simulink model "mdl4_20160413_004644"  (R2014a)
settings: Solver=FixedStepDiscrete  SolverMode=SingleTasking  StartTime=TIME(1)  StopTime=TIME(end)  FixedStep=SIMSTEP  RelTol=1e-3
model workspace (MAT data in the model file):
  autoc_mdd_data01 : struct (value not decoded)
undefined symbols (not defined in the file): Parameter113, Parameter131, Parameter132, Parameter144, Parameter51, Parameter52, Parameter53, Parameter54, Parameter69, Parameter91, SIMSTEP
(part 2 of 3)

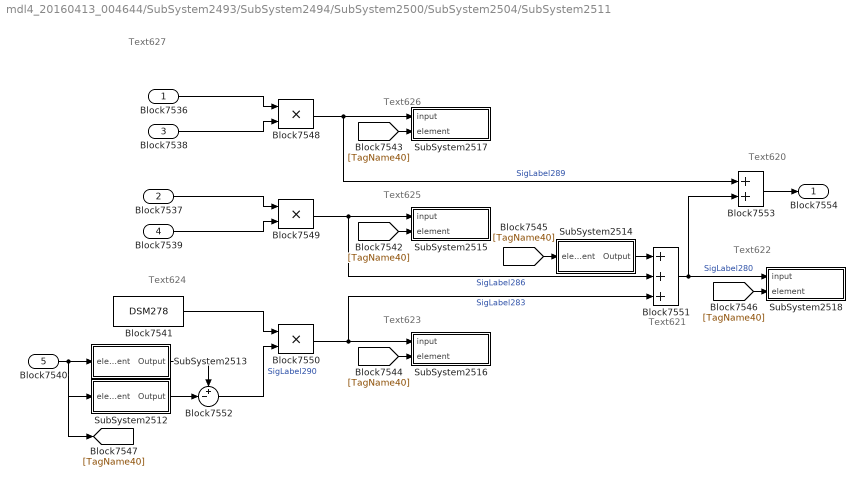
== system mdl4_20160413_004644/SubSystem2493/SubSystem2494/SubSystem2500/SubSystem2504/SubSystem2511 ==
  note: Text627
  note: Text626
  note: Text625
  note: Text624
  note: Text623
  note: Text622
  note: Text621
  note: Text620
  Block7536 : Inport
  Block7537 : Inport  Port=2
  Block7538 : Inport  Port=3
  Block7539 : Inport  Port=4
  Block7540 : Inport  Port=5
  Block7541 : DataStoreRead  DataStoreName=DSM278
  Block7548 : Product  OutDataTypeStr=double  SaturateOnIntegerOverflow=on  RndMeth=Zero  InputSameDT=on
  Block7549 : Product  OutDataTypeStr=double  SaturateOnIntegerOverflow=on  RndMeth=Zero  InputSameDT=on
  Block7550 : Product  OutDataTypeStr=double  SaturateOnIntegerOverflow=on  RndMeth=Zero  InputSameDT=on
  Block7551 : Sum  Inputs=3  OutDataTypeStr=double  RndMeth=Zero  SaturateOnIntegerOverflow=on  InputSameDT=on
  Block7552 : Sum  Inputs=+-|  OutDataTypeStr=double  RndMeth=Zero  SaturateOnIntegerOverflow=on  InputSameDT=on
  Block7553 : Sum  Inputs=2  OutDataTypeStr=double  RndMeth=Zero  SaturateOnIntegerOverflow=on  InputSameDT=on
  SubSystem2512 : Subsystem  TreatAsAtomicUnit=on  mask(***ATC.DSRVEC***){bd_version=1.01.A, r0=DSM258, r1=-1, r2=, r3=, r4=, r5=, r6=, r7=, r8=, r9=, c0=, c1=, c2=, c3=, c4=, c5=, c6=, c7=, c8=, c9=}
      mask prompts: bd_version "Version"
      mask help: これはAutoCからのブロックです．編集禁止．
      settings: OpenFcn=warndlg('変更禁止!');
      mask Help: web(ui_blockhelpmng(gcb));
      mask Display: disp('ATC.DSRVEC')
  SubSystem2513 : Subsystem  TreatAsAtomicUnit=on  mask(***ATC.DSRVEC***){bd_version=1.01.A, r0=DSM259, r1=-1, r2=, r3=, r4=, r5=, r6=, r7=, r8=, r9=, c0=, c1=, c2=, c3=, c4=, c5=, c6=, c7=, c8=, c9=}
      mask prompts: bd_version "Version"
      mask help: これはAutoCからのブロックです．編集禁止．
      settings: OpenFcn=warndlg('変更禁止!');
      mask Help: web(ui_blockhelpmng(gcb));
      mask Display: disp('ATC.DSRVEC')
  SubSystem2514 : Subsystem  TreatAsAtomicUnit=on  mask(***ATC.DSRVEC***){bd_version=1.01.A, r0=DSM300, r1=-1, r2=, r3=, r4=, r5=, r6=, r7=, r8=, r9=, c0=, c1=, c2=, c3=, c4=, c5=, c6=, c7=, c8=, c9=}
      mask prompts: bd_version "Version"
      mask help: これはAutoCからのブロックです．編集禁止．
      settings: OpenFcn=warndlg('変更禁止!');
      mask Help: web(ui_blockhelpmng(gcb));
      mask Display: disp('ATC.DSRVEC')
  SubSystem2515 : Subsystem  TreatAsAtomicUnit=on  mask(***ATC.DSWVEC***){bd_version=1.01.A, r0=DSM302, r1=-1, r2=, r3=, r4=, r5=, r6=, r7=, r8=, r9=, c0=, c1=, c2=, c3=, c4=, c5=, c6=, c7=, c8=, c9=}
      mask prompts: bd_version "Version"
      mask help: これはAutoCからのブロックです．編集禁止．
      settings: OpenFcn=warndlg('変更禁止!');
      mask Help: web(ui_blockhelpmng(gcb));
      mask Display: disp('ATC.DSRVEC')
  SubSystem2516 : Subsystem  TreatAsAtomicUnit=on  mask(***ATC.DSWVEC***){bd_version=1.01.A, r0=DSM301, r1=-1, r2=, r3=, r4=, r5=, r6=, r7=, r8=, r9=, c0=, c1=, c2=, c3=, c4=, c5=, c6=, c7=, c8=, c9=}
      mask prompts: bd_version "Version"
      mask help: これはAutoCからのブロックです．編集禁止．
      settings: OpenFcn=warndlg('変更禁止!');
      mask Help: web(ui_blockhelpmng(gcb));
      mask Display: disp('ATC.DSRVEC')
  SubSystem2517 : Subsystem  TreatAsAtomicUnit=on  mask(***ATC.DSWVEC***){bd_version=1.01.A, r0=DSM303, r1=-1, r2=, r3=, r4=, r5=, r6=, r7=, r8=, r9=, c0=, c1=, c2=, c3=, c4=, c5=, c6=, c7=, c8=, c9=}
      mask prompts: bd_version "Version"
      mask help: これはAutoCからのブロックです．編集禁止．
      settings: OpenFcn=warndlg('変更禁止!');
      mask Help: web(ui_blockhelpmng(gcb));
      mask Display: disp('ATC.DSRVEC')
  SubSystem2518 : Subsystem  TreatAsAtomicUnit=on  mask(***ATC.DSWVEC***){bd_version=1.01.A, r0=DSM300, r1=-1, r2=, r3=, r4=, r5=, r6=, r7=, r8=, r9=, c0=, c1=, c2=, c3=, c4=, c5=, c6=, c7=, c8=, c9=}
      mask prompts: bd_version "Version"
      mask help: これはAutoCからのブロックです．編集禁止．
      settings: OpenFcn=warndlg('変更禁止!');
      mask Help: web(ui_blockhelpmng(gcb));
      mask Display: disp('ATC.DSRVEC')
  Block7554 : Outport
  wires:
  SubSystem2512/1(Output) -> Block7552/2
  SubSystem2513/1(Output) -> Block7552/1
  Block7540/1 -> SubSystem2513/1(element), SubSystem2512/1(element), [TagName40]
  Block7552/1 -> Block7550/2  "SigLabel290"
  Block7548/1 -> SubSystem2517/1(input), Block7553/1  "SigLabel289"
  [TagName40] -> SubSystem2517/2(element)
  Block7549/1 -> SubSystem2515/1(input), Block7551/2  "SigLabel286"
  [TagName40] -> SubSystem2515/2(element)
  Block7541/1 -> Block7550/1
  Block7550/1 -> SubSystem2516/1(input), Block7551/3  "SigLabel283"
  [TagName40] -> SubSystem2516/2(element)
  [TagName40] -> SubSystem2514/1(element)
  [TagName40] -> SubSystem2518/2(element)
  SubSystem2514/1(Output) -> Block7551/1
  Block7551/1 -> SubSystem2518/1(input), Block7553/2  "SigLabel280"
  Block7553/1 -> Block7554/1
  Block7536/1 -> Block7548/1
  Block7538/1 -> Block7548/2
  Block7537/1 -> Block7549/1
  Block7539/1 -> Block7549/2

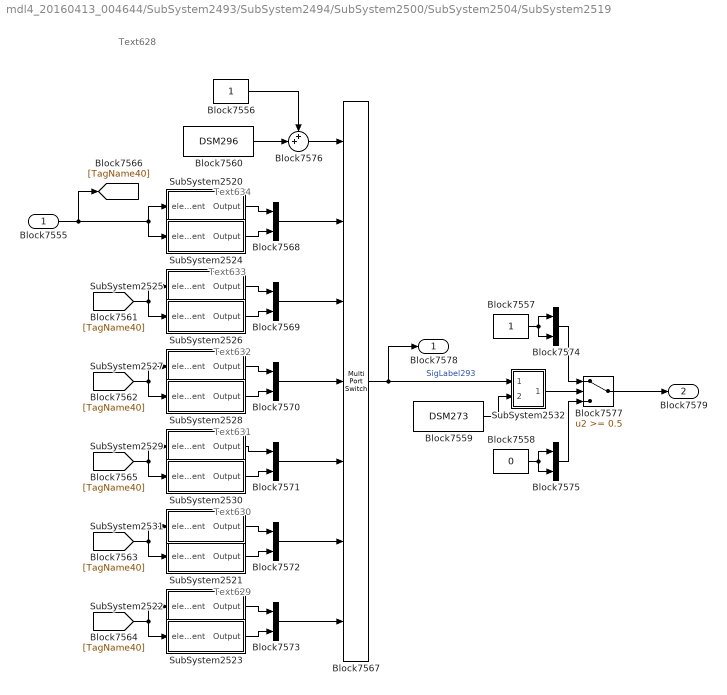
== system mdl4_20160413_004644/SubSystem2493/SubSystem2494/SubSystem2500/SubSystem2504/SubSystem2519 ==
  note: Text634
  note: Text633
  note: Text632
  note: Text631
  note: Text630
  note: Text629
  note: Text628
  Block7555 : Inport
  Block7556 : Constant  OutDataTypeStr=double  SampleTime=-1
  Block7557 : Constant  OutDataTypeStr=double  SampleTime=-1
  Block7558 : Constant  Value=0  OutDataTypeStr=double  SampleTime=-1
  Block7559 : DataStoreRead  DataStoreName=DSM273
  Block7560 : DataStoreRead  DataStoreName=DSM296
  Block7567 : MultiPortSwitch  Inputs=6  RndMeth=Zero  SaturateOnIntegerOverflow=on  InputSameDT=on
  Block{7568..7575} (8 alike) : Mux  Inputs=2
  Block7576 : Sum  Inputs=++|  OutDataTypeStr=double  RndMeth=Zero  SaturateOnIntegerOverflow=on  InputSameDT=on
  Block7577 : Switch  Threshold=0.5  RndMeth=Zero  SaturateOnIntegerOverflow=on  InputSameDT=on
  SubSystem2520 : Subsystem  TreatAsAtomicUnit=on  mask(***ATC.DSRVEC***){bd_version=1.01.A, r0=DSM114, r1=-1, r2=, r3=, r4=, r5=, r6=, r7=, r8=, r9=, c0=, c1=, c2=, c3=, c4=, c5=, c6=, c7=, c8=, c9=}
      mask prompts: bd_version "Version"
      mask help: これはAutoCからのブロックです．編集禁止．
      settings: OpenFcn=warndlg('変更禁止!');
      mask Help: web(ui_blockhelpmng(gcb));
      mask Display: disp('ATC.DSRVEC')
  SubSystem2521 : Subsystem  TreatAsAtomicUnit=on  mask(***ATC.DSRVEC***){bd_version=1.01.A, r0=DSM105, r1=-1, r2=, r3=, r4=, r5=, r6=, r7=, r8=, r9=, c0=, c1=, c2=, c3=, c4=, c5=, c6=, c7=, c8=, c9=}
      mask prompts: bd_version "Version"
      mask help: これはAutoCからのブロックです．編集禁止．
      settings: OpenFcn=warndlg('変更禁止!');
      mask Help: web(ui_blockhelpmng(gcb));
      mask Display: disp('ATC.DSRVEC')
  SubSystem2522 : Subsystem  TreatAsAtomicUnit=on  mask(***ATC.DSRVEC***){bd_version=1.01.A, r0=DSM111, r1=-1, r2=, r3=, r4=, r5=, r6=, r7=, r8=, r9=, c0=, c1=, c2=, c3=, c4=, c5=, c6=, c7=, c8=, c9=}
      mask prompts: bd_version "Version"
      mask help: これはAutoCからのブロックです．編集禁止．
      settings: OpenFcn=warndlg('変更禁止!');
      mask Help: web(ui_blockhelpmng(gcb));
      mask Display: disp('ATC.DSRVEC')
  SubSystem2523 : Subsystem  TreatAsAtomicUnit=on  mask(***ATC.DSRVEC***){bd_version=1.01.A, r0=DSM113, r1=-1, r2=, r3=, r4=, r5=, r6=, r7=, r8=, r9=, c0=, c1=, c2=, c3=, c4=, c5=, c6=, c7=, c8=, c9=}
      mask prompts: bd_version "Version"
      mask help: これはAutoCからのブロックです．編集禁止．
      settings: OpenFcn=warndlg('変更禁止!');
      mask Help: web(ui_blockhelpmng(gcb));
      mask Display: disp('ATC.DSRVEC')
  SubSystem2524 : Subsystem  TreatAsAtomicUnit=on  mask(***ATC.DSRVEC***){bd_version=1.01.A, r0=DSM118, r1=-1, r2=, r3=, r4=, r5=, r6=, r7=, r8=, r9=, c0=, c1=, c2=, c3=, c4=, c5=, c6=, c7=, c8=, c9=}
      mask prompts: bd_version "Version"
      mask help: これはAutoCからのブロックです．編集禁止．
      settings: OpenFcn=warndlg('変更禁止!');
      mask Help: web(ui_blockhelpmng(gcb));
      mask Display: disp('ATC.DSRVEC')
  SubSystem2525 : Subsystem  TreatAsAtomicUnit=on  mask(***ATC.DSRVEC***){bd_version=1.01.A, r0=DSM117, r1=-1, r2=, r3=, r4=, r5=, r6=, r7=, r8=, r9=, c0=, c1=, c2=, c3=, c4=, c5=, c6=, c7=, c8=, c9=}
      mask prompts: bd_version "Version"
      mask help: これはAutoCからのブロックです．編集禁止．
      settings: OpenFcn=warndlg('変更禁止!');
      mask Help: web(ui_blockhelpmng(gcb));
      mask Display: disp('ATC.DSRVEC')
  SubSystem2526 : Subsystem  TreatAsAtomicUnit=on  mask(***ATC.DSRVEC***){bd_version=1.01.A, r0=DSM121, r1=-1, r2=, r3=, r4=, r5=, r6=, r7=, r8=, r9=, c0=, c1=, c2=, c3=, c4=, c5=, c6=, c7=, c8=, c9=}
      mask prompts: bd_version "Version"
      mask help: これはAutoCからのブロックです．編集禁止．
      settings: OpenFcn=warndlg('変更禁止!');
      mask Help: web(ui_blockhelpmng(gcb));
      mask Display: disp('ATC.DSRVEC')
  SubSystem2527 : Subsystem  TreatAsAtomicUnit=on  mask(***ATC.DSRVEC***){bd_version=1.01.A, r0=DSM124, r1=-1, r2=, r3=, r4=, r5=, r6=, r7=, r8=, r9=, c0=, c1=, c2=, c3=, c4=, c5=, c6=, c7=, c8=, c9=}
      mask prompts: bd_version "Version"
      mask help: これはAutoCからのブロックです．編集禁止．
      settings: OpenFcn=warndlg('変更禁止!');
      mask Help: web(ui_blockhelpmng(gcb));
      mask Display: disp('ATC.DSRVEC')
  SubSystem2528 : Subsystem  TreatAsAtomicUnit=on  mask(***ATC.DSRVEC***){bd_version=1.01.A, r0=DSM127, r1=-1, r2=, r3=, r4=, r5=, r6=, r7=, r8=, r9=, c0=, c1=, c2=, c3=, c4=, c5=, c6=, c7=, c8=, c9=}
      mask prompts: bd_version "Version"
      mask help: これはAutoCからのブロックです．編集禁止．
      settings: OpenFcn=warndlg('変更禁止!');
      mask Help: web(ui_blockhelpmng(gcb));
      mask Display: disp('ATC.DSRVEC')
  SubSystem2529 : Subsystem  TreatAsAtomicUnit=on  mask(***ATC.DSRVEC***){bd_version=1.01.A, r0=DSM107, r1=-1, r2=, r3=, r4=, r5=, r6=, r7=, r8=, r9=, c0=, c1=, c2=, c3=, c4=, c5=, c6=, c7=, c8=, c9=}
      mask prompts: bd_version "Version"
      mask help: これはAutoCからのブロックです．編集禁止．
      settings: OpenFcn=warndlg('変更禁止!');
      mask Help: web(ui_blockhelpmng(gcb));
      mask Display: disp('ATC.DSRVEC')
  SubSystem2530 : Subsystem  TreatAsAtomicUnit=on  mask(***ATC.DSRVEC***){bd_version=1.01.A, r0=DSM109, r1=-1, r2=, r3=, r4=, r5=, r6=, r7=, r8=, r9=, c0=, c1=, c2=, c3=, c4=, c5=, c6=, c7=, c8=, c9=}
      mask prompts: bd_version "Version"
      mask help: これはAutoCからのブロックです．編集禁止．
      settings: OpenFcn=warndlg('変更禁止!');
      mask Help: web(ui_blockhelpmng(gcb));
      mask Display: disp('ATC.DSRVEC')
  SubSystem2531 : Subsystem  TreatAsAtomicUnit=on  mask(***ATC.DSRVEC***){bd_version=1.01.A, r0=DSM103, r1=-1, r2=, r3=, r4=, r5=, r6=, r7=, r8=, r9=, c0=, c1=, c2=, c3=, c4=, c5=, c6=, c7=, c8=, c9=}
      mask prompts: bd_version "Version"
      mask help: これはAutoCからのブロックです．編集禁止．
      settings: OpenFcn=warndlg('変更禁止!');
      mask Help: web(ui_blockhelpmng(gcb));
      mask Display: disp('ATC.DSRVEC')
  SubSystem2532 : Subsystem
  Block7578 : Outport
  Block7579 : Outport  Port=2
  wires:
  Block7560/1 -> Block7576/2
  Block7556/1 -> Block7576/1
  Block7576/1 -> Block7567/1
  Block7555/1 -> SubSystem2524/1(element), SubSystem2520/1(element), [TagName40]
  SubSystem2520/1(Output) -> Block7568/1
  SubSystem2524/1(Output) -> Block7568/2
  Block7568/1 -> Block7567/2
  [TagName40] -> SubSystem2525/1(element), SubSystem2526/1(element)
  SubSystem2525/1(Output) -> Block7569/1
  SubSystem2526/1(Output) -> Block7569/2
  [TagName40] -> SubSystem2527/1(element), SubSystem2528/1(element)
  SubSystem2527/1(Output) -> Block7570/1
  SubSystem2528/1(Output) -> Block7570/2
  [TagName40] -> SubSystem2529/1(element), SubSystem2530/1(element)
  SubSystem2530/1(Output) -> Block7571/2
  [TagName40] -> SubSystem2531/1(element), SubSystem2521/1(element)
  SubSystem2531/1(Output) -> Block7572/1
  SubSystem2521/1(Output) -> Block7572/2
  [TagName40] -> SubSystem2522/1(element), SubSystem2523/1(element)
  SubSystem2522/1(Output) -> Block7573/1
  SubSystem2523/1(Output) -> Block7573/2
  SubSystem2529/1(Output) -> Block7571/1
  Block7569/1 -> Block7567/3
  Block7570/1 -> Block7567/4
  Block7571/1 -> Block7567/5
  Block7572/1 -> Block7567/6
  Block7573/1 -> Block7567/7
  Block7567/1 -> Block7578/1, SubSystem2532/1(In1)  "SigLabel293"
  Block7559/1 -> SubSystem2532/2(In2)
  SubSystem2532/1(Out1) -> Block7577/2
  Block7577/1 -> Block7579/1
  Block7557/1 -> Block7574/1, Block7574/2
  Block7558/1 -> Block7575/1, Block7575/2
  Block7574/1 -> Block7577/1
  Block7575/1 -> Block7577/3

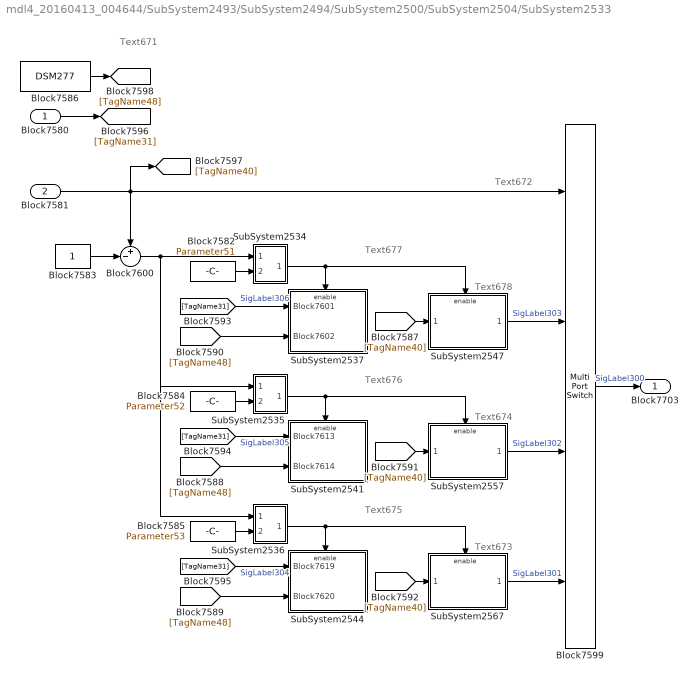
== system mdl4_20160413_004644/SubSystem2493/SubSystem2494/SubSystem2500/SubSystem2504/SubSystem2533 ==
  note: Text678
  note: Text677
  note: Text676
  note: Text675
  note: Text674
  note: Text673
  note: Text672
  note: Text671
  Block7580 : Inport
  Block7581 : Inport  Port=2
  Block7582 : Constant  Value=Parameter51  OutDataTypeStr=double  SampleTime=-1
  Block7583 : Constant  OutDataTypeStr=double  SampleTime=-1
  Block7584 : Constant  Value=Parameter52  OutDataTypeStr=double  SampleTime=-1
  Block7585 : Constant  Value=Parameter53  OutDataTypeStr=double  SampleTime=-1
  Block7586 : DataStoreRead  DataStoreName=DSM277
  Block7599 : MultiPortSwitch  RndMeth=Zero  SaturateOnIntegerOverflow=on  InputSameDT=on
  Block7600 : Sum  Inputs=+-|  OutDataTypeStr=double  RndMeth=Zero  SaturateOnIntegerOverflow=on  InputSameDT=on
  SubSystem2534 : Subsystem
  SubSystem2535 : Subsystem
  SubSystem2536 : Subsystem
  SubSystem2537 : Subsystem  Priority=10  TreatAsAtomicUnit=on
      settings: AttributesFormatString=Attribute1933
  SubSystem2541 : Subsystem  Priority=10  TreatAsAtomicUnit=on
      settings: AttributesFormatString=Attribute1939
  SubSystem2544 : Subsystem  Priority=10  TreatAsAtomicUnit=on
      settings: AttributesFormatString=Attribute1943
  SubSystem2547 : Subsystem  Priority=20  TreatAsAtomicUnit=on
      settings: AttributesFormatString=Attribute1947
  SubSystem2557 : Subsystem  Priority=20  TreatAsAtomicUnit=on
      settings: AttributesFormatString=Attribute1954
  SubSystem2567 : Subsystem  Priority=20  TreatAsAtomicUnit=on
      settings: AttributesFormatString=Attribute1961
  Block7703 : Outport
  wires:
  Block7582/1 -> SubSystem2534/2(In2)
  SubSystem2534/1(Out1) -> SubSystem2537/Enable, SubSystem2547/Enable
  [TagName31] -> SubSystem2537/1(Block7601)  "SigLabel306"
  Block7584/1 -> SubSystem2535/2(In2)
  [TagName48] -> SubSystem2541/2(Block7614)
  SubSystem2535/1(Out1) -> SubSystem2541/Enable, SubSystem2557/Enable
  [TagName31] -> SubSystem2541/1(Block7613)  "SigLabel305"
  Block7585/1 -> SubSystem2536/2(In2)
  [TagName48] -> SubSystem2544/2(Block7620)
  SubSystem2536/1(Out1) -> SubSystem2544/Enable, SubSystem2567/Enable
  [TagName31] -> SubSystem2544/1(Block7619)  "SigLabel304"
  [TagName48] -> SubSystem2537/2(Block7602)
  SubSystem2547/1(Block7650) -> Block7599/2  "SigLabel303"
  SubSystem2557/1(Block7676) -> Block7599/3  "SigLabel302"
  SubSystem2567/1(Block7702) -> Block7599/4  "SigLabel301"
  Block7581/1 -> Block7599/1, Block7600/1, [TagName40]
  Block7599/1 -> Block7703/1  "SigLabel300"
  Block7583/1 -> Block7600/2
  Block7600/1 -> SubSystem2535/1(In1), SubSystem2536/1(In1), SubSystem2534/1(In1)
  Block7586/1 -> [TagName48]
  Block7580/1 -> [TagName31]
  [TagName40] -> SubSystem2547/1(Block7625)
  [TagName40] -> SubSystem2557/1(Block7651)
  [TagName40] -> SubSystem2567/1(Block7677)

== system mdl4_20160413_004644/SubSystem2493/SubSystem2577/SubSystem2579/SubSystem2581/SubSystem2582 ==
  note: ***編集禁止***
  input : Inport
  element : Inport  Port=2
  Assignment : Assignment  IndexOptions=Index vector (port)  OutputSizes=[1 1]
  Inside_DSR : DataStoreRead  DataStoreName=DSM258
  Inside_DSW : DataStoreWrite  DataStoreName=DSM258
  wires:
  Assignment/1 -> Inside_DSW/1
  Inside_DSR/1 -> Assignment/1
  input/1 -> Assignment/2
  element/1 -> Assignment/3

== system mdl4_20160413_004644/SubSystem2493/SubSystem2577/SubSystem2579/SubSystem2581/SubSystem2583 ==
  note: ***編集禁止***
  input : Inport
  element : Inport  Port=2
  Assignment : Assignment  IndexOptions=Index vector (port)  OutputSizes=[1 1]
  Inside_DSR : DataStoreRead  DataStoreName=DSM275
  Inside_DSW : DataStoreWrite  DataStoreName=DSM275
  wires:
  Assignment/1 -> Inside_DSW/1
  Inside_DSR/1 -> Assignment/1
  input/1 -> Assignment/2
  element/1 -> Assignment/3

== system mdl4_20160413_004644/SubSystem2493/SubSystem2577/SubSystem2579/SubSystem2581/SubSystem2584 ==
  note: ***編集禁止***
  input : Inport
  element : Inport  Port=2
  Assignment : Assignment  IndexOptions=Index vector (port)  OutputSizes=[1 1]
  Inside_DSR : DataStoreRead  DataStoreName=DSM295
  Inside_DSW : DataStoreWrite  DataStoreName=DSM295
  wires:
  Assignment/1 -> Inside_DSW/1
  Inside_DSR/1 -> Assignment/1
  input/1 -> Assignment/2
  element/1 -> Assignment/3

== system mdl4_20160413_004644/SubSystem2493/SubSystem2577/SubSystem2579/SubSystem2581/SubSystem2585 ==
  note: ***編集禁止***
  input : Inport
  element : Inport  Port=2
  Assignment : Assignment  IndexOptions=Index vector (port)  OutputSizes=[1 1]
  Inside_DSR : DataStoreRead  DataStoreName=DSM280
  Inside_DSW : DataStoreWrite  DataStoreName=DSM280
  wires:
  Assignment/1 -> Inside_DSW/1
  Inside_DSR/1 -> Assignment/1
  input/1 -> Assignment/2
  element/1 -> Assignment/3

== system mdl4_20160413_004644/SubSystem2493/SubSystem2577/SubSystem2579/SubSystem2581/SubSystem2586 ==
  note: ***編集禁止***
  input : Inport
  element : Inport  Port=2
  Assignment : Assignment  IndexOptions=Index vector (port)  OutputSizes=[1 1]
  Inside_DSR : DataStoreRead  DataStoreName=DSM282
  Inside_DSW : DataStoreWrite  DataStoreName=DSM282
  wires:
  Assignment/1 -> Inside_DSW/1
  Inside_DSR/1 -> Assignment/1
  input/1 -> Assignment/2
  element/1 -> Assignment/3

== system mdl4_20160413_004644/SubSystem2493/SubSystem2577/SubSystem2579/SubSystem2581/SubSystem2587 ==
  note: ***編集禁止***
  input : Inport
  element : Inport  Port=2
  Assignment : Assignment  IndexOptions=Index vector (port)  OutputSizes=[1 1]
  Inside_DSR : DataStoreRead  DataStoreName=DSM274
  Inside_DSW : DataStoreWrite  DataStoreName=DSM274
  wires:
  Assignment/1 -> Inside_DSW/1
  Inside_DSR/1 -> Assignment/1
  input/1 -> Assignment/2
  element/1 -> Assignment/3

== system mdl4_20160413_004644/SubSystem2493/SubSystem2577/SubSystem2579/SubSystem2581/SubSystem2588 ==
  note: ***編集禁止***
  input : Inport
  element : Inport  Port=2
  Assignment : Assignment  IndexOptions=Index vector (port)  OutputSizes=[1 1]
  Inside_DSR : DataStoreRead  DataStoreName=DSM302
  Inside_DSW : DataStoreWrite  DataStoreName=DSM302
  wires:
  Assignment/1 -> Inside_DSW/1
  Inside_DSR/1 -> Assignment/1
  input/1 -> Assignment/2
  element/1 -> Assignment/3

== system mdl4_20160413_004644/SubSystem2493/SubSystem2577/SubSystem2579/SubSystem2581/SubSystem2589 ==
  note: ***編集禁止***
  input : Inport
  element : Inport  Port=2
  Assignment : Assignment  IndexOptions=Index vector (port)  OutputSizes=[1 1]
  Inside_DSR : DataStoreRead  DataStoreName=DSM303
  Inside_DSW : DataStoreWrite  DataStoreName=DSM303
  wires:
  Assignment/1 -> Inside_DSW/1
  Inside_DSR/1 -> Assignment/1
  input/1 -> Assignment/2
  element/1 -> Assignment/3

== system mdl4_20160413_004644/SubSystem2493/SubSystem2577/SubSystem2579/SubSystem2581/SubSystem2590 ==
  note: ***編集禁止***
  input : Inport
  element : Inport  Port=2
  Assignment : Assignment  IndexOptions=Index vector (port)  OutputSizes=[1 1]
  Inside_DSR : DataStoreRead  DataStoreName=DSM300
  Inside_DSW : DataStoreWrite  DataStoreName=DSM300
  wires:
  Assignment/1 -> Inside_DSW/1
  Inside_DSR/1 -> Assignment/1
  input/1 -> Assignment/2
  element/1 -> Assignment/3

== system mdl4_20160413_004644/SubSystem2493/SubSystem2577/SubSystem2579/SubSystem2581/SubSystem2591 ==
  note: ***編集禁止***
  input : Inport
  element : Inport  Port=2
  Assignment : Assignment  IndexOptions=Index vector (port)  OutputSizes=[1 1]
  Inside_DSR : DataStoreRead  DataStoreName=DSM301
  Inside_DSW : DataStoreWrite  DataStoreName=DSM301
  wires:
  Assignment/1 -> Inside_DSW/1
  Inside_DSR/1 -> Assignment/1
  input/1 -> Assignment/2
  element/1 -> Assignment/3

== system mdl4_20160413_004644/SubSystem2493/SubSystem2577/SubSystem2579/SubSystem2581/SubSystem2592 ==
  note: ***編集禁止***
  input : Inport
  element : Inport  Port=2
  Assignment : Assignment  IndexOptions=Index vector (port)  OutputSizes=[1 1]
  Inside_DSR : DataStoreRead  DataStoreName=DSM293
  Inside_DSW : DataStoreWrite  DataStoreName=DSM293
  wires:
  Assignment/1 -> Inside_DSW/1
  Inside_DSR/1 -> Assignment/1
  input/1 -> Assignment/2
  element/1 -> Assignment/3

== system mdl4_20160413_004644/SubSystem2493/SubSystem2577/SubSystem2579/SubSystem2581/SubSystem2593 ==
  note: ***編集禁止***
  input : Inport
  element : Inport  Port=2
  Assignment : Assignment  IndexOptions=Index vector (port)  OutputSizes=[1 1]
  Inside_DSR : DataStoreRead  DataStoreName=DSM279
  Inside_DSW : DataStoreWrite  DataStoreName=DSM279
  wires:
  Assignment/1 -> Inside_DSW/1
  Inside_DSR/1 -> Assignment/1
  input/1 -> Assignment/2
  element/1 -> Assignment/3

== system mdl4_20160413_004644/SubSystem2493/SubSystem2577/SubSystem2579/SubSystem2581/SubSystem2594 ==
  note: ***編集禁止***
  input : Inport
  element : Inport  Port=2
  Assignment : Assignment  IndexOptions=Index vector (port)  OutputSizes=[1 1]
  Inside_DSR : DataStoreRead  DataStoreName=DSM281
  Inside_DSW : DataStoreWrite  DataStoreName=DSM281
  wires:
  Assignment/1 -> Inside_DSW/1
  Inside_DSR/1 -> Assignment/1
  input/1 -> Assignment/2
  element/1 -> Assignment/3

== system mdl4_20160413_004644/SubSystem2493/SubSystem2494/SubSystem2500/SubSystem2504/SubSystem2507/SubSystem2508 ==
  note: ***編集禁止***
  In1 : Inport
  In2 : Inport  Port=2
  RO1 : RelationalOperator  Operator===  InputSameDT=on
  single1 : DataTypeConversion  OutDataTypeStr=single  SaturateOnIntegerOverflow=on  RndMeth=Zero
  single2 : DataTypeConversion  OutDataTypeStr=single  SaturateOnIntegerOverflow=on  RndMeth=Zero
  Out1 : Outport
  wires:
  RO1/1 -> Out1/1
  In2/1 -> single2/1
  In1/1 -> single1/1
  single1/1 -> RO1/1
  single2/1 -> RO1/2

== system mdl4_20160413_004644/SubSystem2493/SubSystem2494/SubSystem2500/SubSystem2504/SubSystem2509/SubSystem2510 ==
  note: ***編集禁止***
  In1 : Inport
  In2 : Inport  Port=2
  RO1 : RelationalOperator  Operator===  InputSameDT=on
  single1 : DataTypeConversion  OutDataTypeStr=single  SaturateOnIntegerOverflow=on  RndMeth=Zero
  single2 : DataTypeConversion  OutDataTypeStr=single  SaturateOnIntegerOverflow=on  RndMeth=Zero
  Out1 : Outport
  wires:
  single2/1 -> RO1/2
  single1/1 -> RO1/1
  In1/1 -> single1/1
  In2/1 -> single2/1
  RO1/1 -> Out1/1

== system mdl4_20160413_004644/SubSystem2493/SubSystem2494/SubSystem2500/SubSystem2504/SubSystem2511/SubSystem2512 ==
  note: ***編集禁止***
  element : Inport
  Inside_DSR : DataStoreRead  DataStoreName=DSM258
  Selector : Selector  IndexOptions=Index vector (port)  Indices=[1 3]
  Output : Outport
  wires:
  Inside_DSR/1 -> Selector/1
  element/1 -> Selector/2
  Selector/1 -> Output/1

== system mdl4_20160413_004644/SubSystem2493/SubSystem2494/SubSystem2500/SubSystem2504/SubSystem2511/SubSystem2513 ==
  note: ***編集禁止***
  element : Inport
  Inside_DSR : DataStoreRead  DataStoreName=DSM259
  Selector : Selector  IndexOptions=Index vector (port)  Indices=[1 3]
  Output : Outport
  wires:
  Selector/1 -> Output/1
  element/1 -> Selector/2
  Inside_DSR/1 -> Selector/1

== system mdl4_20160413_004644/SubSystem2493/SubSystem2494/SubSystem2500/SubSystem2504/SubSystem2511/SubSystem2514 ==
  note: ***編集禁止***
  element : Inport
  Inside_DSR : DataStoreRead  DataStoreName=DSM300
  Selector : Selector  IndexOptions=Index vector (port)  Indices=[1 3]
  Output : Outport
  wires:
  Inside_DSR/1 -> Selector/1
  element/1 -> Selector/2
  Selector/1 -> Output/1

== system mdl4_20160413_004644/SubSystem2493/SubSystem2494/SubSystem2500/SubSystem2504/SubSystem2511/SubSystem2515 ==
  note: ***編集禁止***
  input : Inport
  element : Inport  Port=2
  Assignment : Assignment  IndexOptions=Index vector (port)  OutputSizes=[1 1]
  Inside_DSR : DataStoreRead  DataStoreName=DSM302
  Inside_DSW : DataStoreWrite  DataStoreName=DSM302
  wires:
  element/1 -> Assignment/3
  input/1 -> Assignment/2
  Inside_DSR/1 -> Assignment/1
  Assignment/1 -> Inside_DSW/1

== system mdl4_20160413_004644/SubSystem2493/SubSystem2494/SubSystem2500/SubSystem2504/SubSystem2511/SubSystem2516 ==
  note: ***編集禁止***
  input : Inport
  element : Inport  Port=2
  Assignment : Assignment  IndexOptions=Index vector (port)  OutputSizes=[1 1]
  Inside_DSR : DataStoreRead  DataStoreName=DSM301
  Inside_DSW : DataStoreWrite  DataStoreName=DSM301
  wires:
  Assignment/1 -> Inside_DSW/1
  Inside_DSR/1 -> Assignment/1
  input/1 -> Assignment/2
  element/1 -> Assignment/3

== system mdl4_20160413_004644/SubSystem2493/SubSystem2494/SubSystem2500/SubSystem2504/SubSystem2511/SubSystem2517 ==
  note: ***編集禁止***
  input : Inport
  element : Inport  Port=2
  Assignment : Assignment  IndexOptions=Index vector (port)  OutputSizes=[1 1]
  Inside_DSR : DataStoreRead  DataStoreName=DSM303
  Inside_DSW : DataStoreWrite  DataStoreName=DSM303
  wires:
  Assignment/1 -> Inside_DSW/1
  Inside_DSR/1 -> Assignment/1
  input/1 -> Assignment/2
  element/1 -> Assignment/3

== system mdl4_20160413_004644/SubSystem2493/SubSystem2494/SubSystem2500/SubSystem2504/SubSystem2511/SubSystem2518 ==
  note: ***編集禁止***
  input : Inport
  element : Inport  Port=2
  Assignment : Assignment  IndexOptions=Index vector (port)  OutputSizes=[1 1]
  Inside_DSR : DataStoreRead  DataStoreName=DSM300
  Inside_DSW : DataStoreWrite  DataStoreName=DSM300
  wires:
  element/1 -> Assignment/3
  input/1 -> Assignment/2
  Inside_DSR/1 -> Assignment/1
  Assignment/1 -> Inside_DSW/1

== system mdl4_20160413_004644/SubSystem2493/SubSystem2494/SubSystem2500/SubSystem2504/SubSystem2519/SubSystem2520 ==
  note: ***編集禁止***
  element : Inport
  Inside_DSR : DataStoreRead  DataStoreName=DSM114
  Selector : Selector  IndexOptions=Index vector (port)  Indices=[1 3]
  Output : Outport
  wires:
  Inside_DSR/1 -> Selector/1
  element/1 -> Selector/2
  Selector/1 -> Output/1

== system mdl4_20160413_004644/SubSystem2493/SubSystem2494/SubSystem2500/SubSystem2504/SubSystem2519/SubSystem2521 ==
  note: ***編集禁止***
  element : Inport
  Inside_DSR : DataStoreRead  DataStoreName=DSM105
  Selector : Selector  IndexOptions=Index vector (port)  Indices=[1 3]
  Output : Outport
  wires:
  Inside_DSR/1 -> Selector/1
  element/1 -> Selector/2
  Selector/1 -> Output/1

== system mdl4_20160413_004644/SubSystem2493/SubSystem2494/SubSystem2500/SubSystem2504/SubSystem2519/SubSystem2522 ==
  note: ***編集禁止***
  element : Inport
  Inside_DSR : DataStoreRead  DataStoreName=DSM111
  Selector : Selector  IndexOptions=Index vector (port)  Indices=[1 3]
  Output : Outport
  wires:
  Inside_DSR/1 -> Selector/1
  element/1 -> Selector/2
  Selector/1 -> Output/1

== system mdl4_20160413_004644/SubSystem2493/SubSystem2494/SubSystem2500/SubSystem2504/SubSystem2519/SubSystem2523 ==
  note: ***編集禁止***
  element : Inport
  Inside_DSR : DataStoreRead  DataStoreName=DSM113
  Selector : Selector  IndexOptions=Index vector (port)  Indices=[1 3]
  Output : Outport
  wires:
  Inside_DSR/1 -> Selector/1
  element/1 -> Selector/2
  Selector/1 -> Output/1

== system mdl4_20160413_004644/SubSystem2493/SubSystem2494/SubSystem2500/SubSystem2504/SubSystem2519/SubSystem2524 ==
  note: ***編集禁止***
  element : Inport
  Inside_DSR : DataStoreRead  DataStoreName=DSM118
  Selector : Selector  IndexOptions=Index vector (port)  Indices=[1 3]
  Output : Outport
  wires:
  Inside_DSR/1 -> Selector/1
  element/1 -> Selector/2
  Selector/1 -> Output/1

== system mdl4_20160413_004644/SubSystem2493/SubSystem2494/SubSystem2500/SubSystem2504/SubSystem2519/SubSystem2525 ==
  note: ***編集禁止***
  element : Inport
  Inside_DSR : DataStoreRead  DataStoreName=DSM117
  Selector : Selector  IndexOptions=Index vector (port)  Indices=[1 3]
  Output : Outport
  wires:
  Inside_DSR/1 -> Selector/1
  element/1 -> Selector/2
  Selector/1 -> Output/1

== system mdl4_20160413_004644/SubSystem2493/SubSystem2494/SubSystem2500/SubSystem2504/SubSystem2519/SubSystem2526 ==
  note: ***編集禁止***
  element : Inport
  Inside_DSR : DataStoreRead  DataStoreName=DSM121
  Selector : Selector  IndexOptions=Index vector (port)  Indices=[1 3]
  Output : Outport
  wires:
  Inside_DSR/1 -> Selector/1
  element/1 -> Selector/2
  Selector/1 -> Output/1

== system mdl4_20160413_004644/SubSystem2493/SubSystem2494/SubSystem2500/SubSystem2504/SubSystem2519/SubSystem2527 ==
  note: ***編集禁止***
  element : Inport
  Inside_DSR : DataStoreRead  DataStoreName=DSM124
  Selector : Selector  IndexOptions=Index vector (port)  Indices=[1 3]
  Output : Outport
  wires:
  Inside_DSR/1 -> Selector/1
  element/1 -> Selector/2
  Selector/1 -> Output/1

== system mdl4_20160413_004644/SubSystem2493/SubSystem2494/SubSystem2500/SubSystem2504/SubSystem2519/SubSystem2528 ==
  note: ***編集禁止***
  element : Inport
  Inside_DSR : DataStoreRead  DataStoreName=DSM127
  Selector : Selector  IndexOptions=Index vector (port)  Indices=[1 3]
  Output : Outport
  wires:
  Inside_DSR/1 -> Selector/1
  element/1 -> Selector/2
  Selector/1 -> Output/1

== system mdl4_20160413_004644/SubSystem2493/SubSystem2494/SubSystem2500/SubSystem2504/SubSystem2519/SubSystem2529 ==
  note: ***編集禁止***
  element : Inport
  Inside_DSR : DataStoreRead  DataStoreName=DSM107
  Selector : Selector  IndexOptions=Index vector (port)  Indices=[1 3]
  Output : Outport
  wires:
  Inside_DSR/1 -> Selector/1
  element/1 -> Selector/2
  Selector/1 -> Output/1

== system mdl4_20160413_004644/SubSystem2493/SubSystem2494/SubSystem2500/SubSystem2504/SubSystem2519/SubSystem2530 ==
  note: ***編集禁止***
  element : Inport
  Inside_DSR : DataStoreRead  DataStoreName=DSM109
  Selector : Selector  IndexOptions=Index vector (port)  Indices=[1 3]
  Output : Outport
  wires:
  Inside_DSR/1 -> Selector/1
  element/1 -> Selector/2
  Selector/1 -> Output/1

== system mdl4_20160413_004644/SubSystem2493/SubSystem2494/SubSystem2500/SubSystem2504/SubSystem2519/SubSystem2531 ==
  note: ***編集禁止***
  element : Inport
  Inside_DSR : DataStoreRead  DataStoreName=DSM103
  Selector : Selector  IndexOptions=Index vector (port)  Indices=[1 3]
  Output : Outport
  wires:
  Inside_DSR/1 -> Selector/1
  element/1 -> Selector/2
  Selector/1 -> Output/1

== system mdl4_20160413_004644/SubSystem2493/SubSystem2494/SubSystem2500/SubSystem2504/SubSystem2519/SubSystem2532 ==
  note: ***編集禁止***
  In1 : Inport
  In2 : Inport  Port=2
  RO1 : RelationalOperator  Operator=>  InputSameDT=on
  single1 : DataTypeConversion  OutDataTypeStr=single  SaturateOnIntegerOverflow=on  RndMeth=Zero
  single2 : DataTypeConversion  OutDataTypeStr=single  SaturateOnIntegerOverflow=on  RndMeth=Zero
  Out1 : Outport
  wires:
  single2/1 -> RO1/2
  single1/1 -> RO1/1
  In1/1 -> single1/1
  In2/1 -> single2/1
  RO1/1 -> Out1/1

== system mdl4_20160413_004644/SubSystem2493/SubSystem2494/SubSystem2500/SubSystem2504/SubSystem2533/SubSystem2534 ==
  note: ***編集禁止***
  In1 : Inport
  In2 : Inport  Port=2
  RO1 : RelationalOperator  Operator===  InputSameDT=on
  single1 : DataTypeConversion  OutDataTypeStr=single  SaturateOnIntegerOverflow=on  RndMeth=Zero
  single2 : DataTypeConversion  OutDataTypeStr=single  SaturateOnIntegerOverflow=on  RndMeth=Zero
  Out1 : Outport
  wires:
  RO1/1 -> Out1/1
  In2/1 -> single2/1
  In1/1 -> single1/1
  single1/1 -> RO1/1
  single2/1 -> RO1/2

== system mdl4_20160413_004644/SubSystem2493/SubSystem2494/SubSystem2500/SubSystem2504/SubSystem2533/SubSystem2535 ==
  note: ***編集禁止***
  In1 : Inport
  In2 : Inport  Port=2
  RO1 : RelationalOperator  Operator===  InputSameDT=on
  single1 : DataTypeConversion  OutDataTypeStr=single  SaturateOnIntegerOverflow=on  RndMeth=Zero
  single2 : DataTypeConversion  OutDataTypeStr=single  SaturateOnIntegerOverflow=on  RndMeth=Zero
  Out1 : Outport
  wires:
  RO1/1 -> Out1/1
  In2/1 -> single2/1
  In1/1 -> single1/1
  single1/1 -> RO1/1
  single2/1 -> RO1/2

== system mdl4_20160413_004644/SubSystem2493/SubSystem2494/SubSystem2500/SubSystem2504/SubSystem2533/SubSystem2536 ==
  note: ***編集禁止***
  In1 : Inport
  In2 : Inport  Port=2
  RO1 : RelationalOperator  Operator===  InputSameDT=on
  single1 : DataTypeConversion  OutDataTypeStr=single  SaturateOnIntegerOverflow=on  RndMeth=Zero
  single2 : DataTypeConversion  OutDataTypeStr=single  SaturateOnIntegerOverflow=on  RndMeth=Zero
  Out1 : Outport
  wires:
  RO1/1 -> Out1/1
  In2/1 -> single2/1
  In1/1 -> single1/1
  single1/1 -> RO1/1
  single2/1 -> RO1/2

== system mdl4_20160413_004644/SubSystem2493/SubSystem2494/SubSystem2500/SubSystem2504/SubSystem2533/SubSystem2537 ==
  note: Text638
  note: Text637
  note: Text636
  note: Text635
  Block7601 : Inport
  Block7602 : Inport  Port=2
  Block7603 : EnablePort
  Block7604 : Constant  OutDataTypeStr=double  SampleTime=-1
  Block7605 : Constant  Value=0  OutDataTypeStr=double  SampleTime=-1
  Block7606 : Constant  OutDataTypeStr=double  SampleTime=-1
  Block7607 : DataStoreRead  DataStoreName=DSM294
  Block7608 : DataStoreWrite  DataStoreName=DSM277
  Block7609 : Demux  Outputs=2
  Block7610 : Sum  Inputs=|++  OutDataTypeStr=double  RndMeth=Zero  SaturateOnIntegerOverflow=on  InputSameDT=on
  Block7611 : Sum  Inputs=++|  OutDataTypeStr=double  RndMeth=Zero  SaturateOnIntegerOverflow=on  InputSameDT=on
  Block7612 : Switch  Threshold=0.5  RndMeth=Zero  SaturateOnIntegerOverflow=on  InputSameDT=on
  SubSystem2538 : Subsystem  Priority=10  TreatAsAtomicUnit=on  mask(***ATC.DSWVEC***){bd_version=1.01.A, r0=DSM293, r1=-1, r2=, r3=, r4=, r5=, r6=, r7=, r8=, r9=, c0=, c1=, c2=, c3=, c4=, c5=, c6=, c7=, c8=, c9=}
      mask prompts: bd_version "Version"
      mask help: これはAutoCからのブロックです．編集禁止．
      settings: AttributesFormatString=Attribute1937  OpenFcn=warndlg('変更禁止!');
      mask Help: web(ui_blockhelpmng(gcb));
      mask Display: disp('ATC.DSRVEC')
  SubSystem2539 : Subsystem  Priority=10  TreatAsAtomicUnit=on  mask(***ATC.DSWVEC***){bd_version=1.01.A, r0=DSM295, r1=-1, r2=, r3=, r4=, r5=, r6=, r7=, r8=, r9=, c0=, c1=, c2=, c3=, c4=, c5=, c6=, c7=, c8=, c9=}
      mask prompts: bd_version "Version"
      mask help: これはAutoCからのブロックです．編集禁止．
      settings: AttributesFormatString=Attribute1938  OpenFcn=warndlg('変更禁止!');
      mask Help: web(ui_blockhelpmng(gcb));
      mask Display: disp('ATC.DSRVEC')
  SubSystem2540 : Subsystem
  wires:
  Block7602/1 -> Block7610/1, Block7611/2
  Block7601/1 -> Block7609/1
  Block7609/1 -> SubSystem2538/1(input)
  Block7609/2 -> SubSystem2539/1(input)
  Block7604/1 -> Block7610/2
  Block7610/1 -> SubSystem2538/2(element), SubSystem2539/2(element)
  Block7607/1 -> SubSystem2540/2(In2)
  Block7606/1 -> Block7611/1
  SubSystem2540/1(Out1) -> Block7612/2
  Block7612/1 -> Block7608/1
  Block7611/1 -> Block7612/3, SubSystem2540/1(In1)
  Block7605/1 -> Block7612/1

== system mdl4_20160413_004644/SubSystem2493/SubSystem2494/SubSystem2500/SubSystem2504/SubSystem2533/SubSystem2541 ==
  note: Text639
  Block7613 : Inport
  Block7614 : Inport  Port=2
  Block7615 : EnablePort
  Block7616 : Constant  OutDataTypeStr=double  SampleTime=-1
  Block7617 : Demux  Outputs=2
  Block7618 : Sum  Inputs=|++  OutDataTypeStr=double  RndMeth=Zero  SaturateOnIntegerOverflow=on  InputSameDT=on
  SubSystem2542 : Subsystem  Priority=10  TreatAsAtomicUnit=on  mask(***ATC.DSWVEC***){bd_version=1.01.A, r0=DSM279, r1=-1, r2=, r3=, r4=, r5=, r6=, r7=, r8=, r9=, c0=, c1=, c2=, c3=, c4=, c5=, c6=, c7=, c8=, c9=}
      mask prompts: bd_version "Version"
      mask help: これはAutoCからのブロックです．編集禁止．
      settings: AttributesFormatString=Attribute1941  OpenFcn=warndlg('変更禁止!');
      mask Help: web(ui_blockhelpmng(gcb));
      mask Display: disp('ATC.DSRVEC')
  SubSystem2543 : Subsystem  Priority=10  TreatAsAtomicUnit=on  mask(***ATC.DSWVEC***){bd_version=1.01.A, r0=DSM280, r1=-1, r2=, r3=, r4=, r5=, r6=, r7=, r8=, r9=, c0=, c1=, c2=, c3=, c4=, c5=, c6=, c7=, c8=, c9=}
      mask prompts: bd_version "Version"
      mask help: これはAutoCからのブロックです．編集禁止．
      settings: AttributesFormatString=Attribute1942  OpenFcn=warndlg('変更禁止!');
      mask Help: web(ui_blockhelpmng(gcb));
      mask Display: disp('ATC.DSRVEC')
  wires:
  Block7613/1 -> Block7617/1
  Block7617/1 -> SubSystem2542/1(input)
  Block7617/2 -> SubSystem2543/1(input)
  Block7616/1 -> Block7618/2
  Block7614/1 -> Block7618/1
  Block7618/1 -> SubSystem2542/2(element), SubSystem2543/2(element)

== system mdl4_20160413_004644/SubSystem2493/SubSystem2494/SubSystem2500/SubSystem2504/SubSystem2533/SubSystem2544 ==
  note: Text640
  Block7619 : Inport
  Block7620 : Inport  Port=2
  Block7621 : EnablePort
  Block7622 : Constant  OutDataTypeStr=double  SampleTime=-1
  Block7623 : Demux  Outputs=2
  Block7624 : Sum  Inputs=|++  OutDataTypeStr=double  RndMeth=Zero  SaturateOnIntegerOverflow=on  InputSameDT=on
  SubSystem2545 : Subsystem  Priority=10  TreatAsAtomicUnit=on  mask(***ATC.DSWVEC***){bd_version=1.01.A, r0=DSM281, r1=-1, r2=, r3=, r4=, r5=, r6=, r7=, r8=, r9=, c0=, c1=, c2=, c3=, c4=, c5=, c6=, c7=, c8=, c9=}
      mask prompts: bd_version "Version"
      mask help: これはAutoCからのブロックです．編集禁止．
      settings: AttributesFormatString=Attribute1945  OpenFcn=warndlg('変更禁止!');
      mask Help: web(ui_blockhelpmng(gcb));
      mask Display: disp('ATC.DSRVEC')
  SubSystem2546 : Subsystem  Priority=10  TreatAsAtomicUnit=on  mask(***ATC.DSWVEC***){bd_version=1.01.A, r0=DSM282, r1=-1, r2=, r3=, r4=, r5=, r6=, r7=, r8=, r9=, c0=, c1=, c2=, c3=, c4=, c5=, c6=, c7=, c8=, c9=}
      mask prompts: bd_version "Version"
      mask help: これはAutoCからのブロックです．編集禁止．
      settings: AttributesFormatString=Attribute1946  OpenFcn=warndlg('変更禁止!');
      mask Help: web(ui_blockhelpmng(gcb));
      mask Display: disp('ATC.DSRVEC')
  wires:
  Block7619/1 -> Block7623/1
  Block7623/1 -> SubSystem2545/1(input)
  Block7623/2 -> SubSystem2546/1(input)
  Block7622/1 -> Block7624/2
  Block7620/1 -> Block7624/1
  Block7624/1 -> SubSystem2545/2(element), SubSystem2546/2(element)

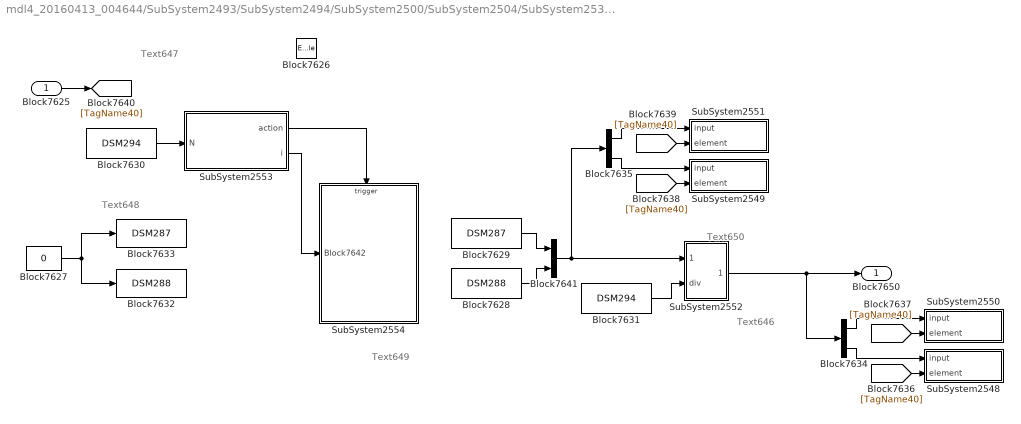
== system mdl4_20160413_004644/SubSystem2493/SubSystem2494/SubSystem2500/SubSystem2504/SubSystem2533/SubSystem2547 ==
  note: Text650
  note: Text649
  note: Text648
  note: Text647
  note: Text646
  Block7625 : Inport
  Block7626 : EnablePort
  Block7627 : Constant  Value=0  OutDataTypeStr=double  SampleTime=-1
  Block7628 : DataStoreRead  Priority=30  DataStoreName=DSM288
      settings: AttributesFormatString=Attribute1949
  Block7629 : DataStoreRead  Priority=30  DataStoreName=DSM287
      settings: AttributesFormatString=Attribute1950
  Block7630 : DataStoreRead  DataStoreName=DSM294
  Block7631 : DataStoreRead  DataStoreName=DSM294
  Block7632 : DataStoreWrite  Priority=10  DataStoreName=DSM288
      settings: AttributesFormatString=Attribute1951
  Block7633 : DataStoreWrite  Priority=10  DataStoreName=DSM287
      settings: AttributesFormatString=Attribute1952
  Block7634 : Demux  Outputs=2
  Block7635 : Demux  Outputs=2
  Block7641 : Mux  Inputs=2
  SubSystem2548 : Subsystem  TreatAsAtomicUnit=on  mask(***ATC.DSWVEC***){bd_version=1.01.A, r0=DSM290, r1=-1, r2=, r3=, r4=, r5=, r6=, r7=, r8=, r9=, c0=, c1=, c2=, c3=, c4=, c5=, c6=, c7=, c8=, c9=}
      mask prompts: bd_version "Version"
      mask help: これはAutoCからのブロックです．編集禁止．
      settings: OpenFcn=warndlg('変更禁止!');
      mask Help: web(ui_blockhelpmng(gcb));
      mask Display: disp('ATC.DSRVEC')
  SubSystem2549 : Subsystem  TreatAsAtomicUnit=on  mask(***ATC.DSWVEC***){bd_version=1.01.A, r0=DSM292, r1=-1, r2=, r3=, r4=, r5=, r6=, r7=, r8=, r9=, c0=, c1=, c2=, c3=, c4=, c5=, c6=, c7=, c8=, c9=}
      mask prompts: bd_version "Version"
      mask help: これはAutoCからのブロックです．編集禁止．
      settings: OpenFcn=warndlg('変更禁止!');
      mask Help: web(ui_blockhelpmng(gcb));
      mask Display: disp('ATC.DSRVEC')
  SubSystem2550 : Subsystem  TreatAsAtomicUnit=on  mask(***ATC.DSWVEC***){bd_version=1.01.A, r0=DSM289, r1=-1, r2=, r3=, r4=, r5=, r6=, r7=, r8=, r9=, c0=, c1=, c2=, c3=, c4=, c5=, c6=, c7=, c8=, c9=}
      mask prompts: bd_version "Version"
      mask help: これはAutoCからのブロックです．編集禁止．
      settings: OpenFcn=warndlg('変更禁止!');
      mask Help: web(ui_blockhelpmng(gcb));
      mask Display: disp('ATC.DSRVEC')
  SubSystem2551 : Subsystem  TreatAsAtomicUnit=on  mask(***ATC.DSWVEC***){bd_version=1.01.A, r0=DSM291, r1=-1, r2=, r3=, r4=, r5=, r6=, r7=, r8=, r9=, c0=, c1=, c2=, c3=, c4=, c5=, c6=, c7=, c8=, c9=}
      mask prompts: bd_version "Version"
      mask help: これはAutoCからのブロックです．編集禁止．
      settings: OpenFcn=warndlg('変更禁止!');
      mask Help: web(ui_blockhelpmng(gcb));
      mask Display: disp('ATC.DSRVEC')
  SubSystem2552 : Subsystem  TreatAsAtomicUnit=on  mask(***ATC.DIVISION***){bd_version=1.01.A, r0=チェック無し, r1=, r2=, r3=, r4=, r5=, r6=, r7=, r8=, r9=, c0=, c1=, c2=, c3=, c4=, c5=, c6=, c7=, c8=, c9=}
      mask prompts: bd_version "Version"
      mask help: これはAutoCからのブロックです．編集禁止．
      settings: OpenFcn=warndlg('変更禁止!');
      mask Help: web(ui_blockhelpmng(gcb));
  SubSystem2553 : Subsystem  Priority=20  TreatAsAtomicUnit=on  mask(***ATC.ITERATOR***){}
      mask help: これはAutoCからのブロックです．編集禁止．
      settings: AttributesFormatString=Attribute1953  OpenFcn=warndlg('変更禁止!');  RTWSystemCode=Inline
  SubSystem2554 : Subsystem  TreatAsAtomicUnit=on
  Block7650 : Outport
  wires:
  Block7627/1 -> Block7632/1, Block7633/1
  Block7635/2 -> SubSystem2549/1(input)
  [TagName40] -> SubSystem2549/2(element)
  Block7635/1 -> SubSystem2551/1(input)
  [TagName40] -> SubSystem2551/2(element)
  Block7634/2 -> SubSystem2548/1(input)
  [TagName40] -> SubSystem2548/2(element)
  Block7634/1 -> SubSystem2550/1(input)
  [TagName40] -> SubSystem2550/2(element)
  Block7641/1 -> Block7635/1, SubSystem2552/1(mult)
  Block7628/1 -> Block7641/2
  Block7629/1 -> Block7641/1
  SubSystem2552/1(Out) -> Block7634/1, Block7650/1
  Block7631/1 -> SubSystem2552/2(div)
  SubSystem2553/2(i) -> SubSystem2554/1(Block7642)
  SubSystem2553/1(action) -> SubSystem2554/Trigger
  Block7630/1 -> SubSystem2553/1(N)
  Block7625/1 -> [TagName40]

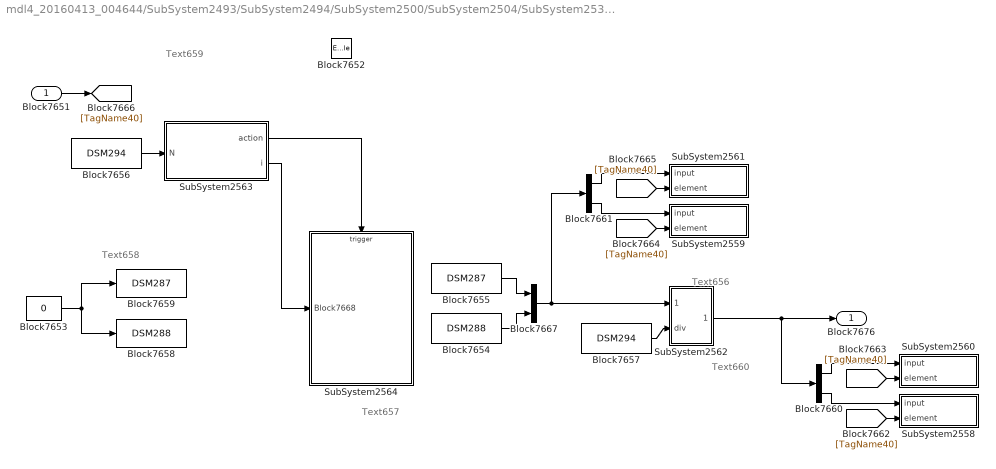
== system mdl4_20160413_004644/SubSystem2493/SubSystem2494/SubSystem2500/SubSystem2504/SubSystem2533/SubSystem2557 ==
  note: Text660
  note: Text659
  note: Text658
  note: Text657
  note: Text656
  Block7651 : Inport
  Block7652 : EnablePort
  Block7653 : Constant  Value=0  OutDataTypeStr=double  SampleTime=-1
  Block7654 : DataStoreRead  Priority=30  DataStoreName=DSM288
      settings: AttributesFormatString=Attribute1956
  Block7655 : DataStoreRead  Priority=30  DataStoreName=DSM287
      settings: AttributesFormatString=Attribute1957
  Block7656 : DataStoreRead  DataStoreName=DSM294
  Block7657 : DataStoreRead  DataStoreName=DSM294
  Block7658 : DataStoreWrite  Priority=10  DataStoreName=DSM288
      settings: AttributesFormatString=Attribute1958
  Block7659 : DataStoreWrite  Priority=10  DataStoreName=DSM287
      settings: AttributesFormatString=Attribute1959
  Block7660 : Demux  Outputs=2
  Block7661 : Demux  Outputs=2
  Block7667 : Mux  Inputs=2
  SubSystem2558 : Subsystem  TreatAsAtomicUnit=on  mask(***ATC.DSWVEC***){bd_version=1.01.A, r0=DSM290, r1=-1, r2=, r3=, r4=, r5=, r6=, r7=, r8=, r9=, c0=, c1=, c2=, c3=, c4=, c5=, c6=, c7=, c8=, c9=}
      mask prompts: bd_version "Version"
      mask help: これはAutoCからのブロックです．編集禁止．
      settings: OpenFcn=warndlg('変更禁止!');
      mask Help: web(ui_blockhelpmng(gcb));
      mask Display: disp('ATC.DSRVEC')
  SubSystem2559 : Subsystem  TreatAsAtomicUnit=on  mask(***ATC.DSWVEC***){bd_version=1.01.A, r0=DSM292, r1=-1, r2=, r3=, r4=, r5=, r6=, r7=, r8=, r9=, c0=, c1=, c2=, c3=, c4=, c5=, c6=, c7=, c8=, c9=}
      mask prompts: bd_version "Version"
      mask help: これはAutoCからのブロックです．編集禁止．
      settings: OpenFcn=warndlg('変更禁止!');
      mask Help: web(ui_blockhelpmng(gcb));
      mask Display: disp('ATC.DSRVEC')
  SubSystem2560 : Subsystem  TreatAsAtomicUnit=on  mask(***ATC.DSWVEC***){bd_version=1.01.A, r0=DSM289, r1=-1, r2=, r3=, r4=, r5=, r6=, r7=, r8=, r9=, c0=, c1=, c2=, c3=, c4=, c5=, c6=, c7=, c8=, c9=}
      mask prompts: bd_version "Version"
      mask help: これはAutoCからのブロックです．編集禁止．
      settings: OpenFcn=warndlg('変更禁止!');
      mask Help: web(ui_blockhelpmng(gcb));
      mask Display: disp('ATC.DSRVEC')
  SubSystem2561 : Subsystem  TreatAsAtomicUnit=on  mask(***ATC.DSWVEC***){bd_version=1.01.A, r0=DSM291, r1=-1, r2=, r3=, r4=, r5=, r6=, r7=, r8=, r9=, c0=, c1=, c2=, c3=, c4=, c5=, c6=, c7=, c8=, c9=}
      mask prompts: bd_version "Version"
      mask help: これはAutoCからのブロックです．編集禁止．
      settings: OpenFcn=warndlg('変更禁止!');
      mask Help: web(ui_blockhelpmng(gcb));
      mask Display: disp('ATC.DSRVEC')
  SubSystem2562 : Subsystem  TreatAsAtomicUnit=on  mask(***ATC.DIVISION***){bd_version=1.01.A, r0=チェック無し, r1=, r2=, r3=, r4=, r5=, r6=, r7=, r8=, r9=, c0=, c1=, c2=, c3=, c4=, c5=, c6=, c7=, c8=, c9=}
      mask prompts: bd_version "Version"
      mask help: これはAutoCからのブロックです．編集禁止．
      settings: OpenFcn=warndlg('変更禁止!');
      mask Help: web(ui_blockhelpmng(gcb));
  SubSystem2563 : Subsystem  Priority=20  TreatAsAtomicUnit=on  mask(***ATC.ITERATOR***){}
      mask help: これはAutoCからのブロックです．編集禁止．
      settings: AttributesFormatString=Attribute1960  OpenFcn=warndlg('変更禁止!');  RTWSystemCode=Inline
  SubSystem2564 : Subsystem  TreatAsAtomicUnit=on
  Block7676 : Outport
  wires:
  Block7656/1 -> SubSystem2563/1(N)
  SubSystem2563/1(action) -> SubSystem2564/Trigger
  SubSystem2563/2(i) -> SubSystem2564/1(Block7668)
  Block7657/1 -> SubSystem2562/2(div)
  SubSystem2562/1(Out) -> Block7676/1, Block7660/1
  Block7655/1 -> Block7667/1
  Block7654/1 -> Block7667/2
  Block7667/1 -> Block7661/1, SubSystem2562/1(mult)
  [TagName40] -> SubSystem2560/2(element)
  Block7660/1 -> SubSystem2560/1(input)
  [TagName40] -> SubSystem2558/2(element)
  Block7660/2 -> SubSystem2558/1(input)
  [TagName40] -> SubSystem2561/2(element)
  Block7661/1 -> SubSystem2561/1(input)
  [TagName40] -> SubSystem2559/2(element)
  Block7661/2 -> SubSystem2559/1(input)
  Block7653/1 -> Block7659/1, Block7658/1
  Block7651/1 -> [TagName40]
